simulink library "PhD_Library"  (R2018a)
settings: Solver=VariableStepAuto  StartTime=0.0  StopTime=10.0  RelTol=1e-3
values from neighbouring files (symbols this model uses):
  Ts = Ts_c    (= 1e-07)    [PlantStateEquations_abc_Script.m]
undefined symbols (not defined in the file or in its folder): D1, Delta, DiscIntNeverNeededParam, ESS, f_LPF_noise, fcutouti, fcutoutv, fn, fsw, Iap, Kp, PCC, Sn, tctrl, Ti, Ts_control, Ts_PWM, Uabp, Uanp, WT, X, zeta
libraries: $bdroot x84, powerlib_meascontrol x59, powerlib x56, peTransforms x32, cstblocks x2, simulink x2
(part 5 of 5)

== matlab function PhD_Library/Offshore_Oil_and_Wind/digital_ramp_gen/MATLAB Function ==
  data: up input; down input; rate input; y output; max input; min input; force input; forceval input; Ts input
%%%%%%%%%%%%%%%%%%%%%%%%%%%%%%%%%%%%%%%%%%%%%%%%%%%%%%%%%%%%%%%%%%%%%%%%%%
% Digital integrator
%%%%%%%%%%%%%%%%%%%%%%%%%%%%%%%%%%%%%%%%%%%%%%%%%%%%%%%%%%%%%%%%%%%%%%%%%%\
% Forward Euler method: as in matlab help
%   y(n) = y(n-1) + Ts(n-1)*x(n-1)
%   uset it to avoid algebraic loops

% All inputs are stored in states, so there is no direct feedthrough
% GAMBIARRA for avoiding algebraic loops
% see: https://www.mathworks.com/help/simulink/ug/integration-considerations-for-matlab-function-blocks.html

% Inputs
%   up: ramps up
%   down: ramps down (if both up and down, than stops)
%   max: max value for ramp
%   min: min value for ramp
%   force: if=1 sets integrator to forceval
%   forceval: see line above (max and min are respected
%   Ts: sampling time
% Output
%   y: output of the ramp

%%%%%%%%%%%%%%%%%%%%%%%%%%%%%%%%%%%%%%%%%%%%%%%%%%%%%%%%%%%%%%%%%%%%%%%%%%\
% Prog/rev history
%   Mota - 2021-05-21: first release

function y = DigRamp(up, down, rate, max, min, force, forceval, Ts)

% The value of the integrator
persistent i
persistent old_up
persistent old_down
persistent old_rate
persistent old_max
persistent old_min
persistent old_force
persistent old_forceval
persistent old_Ts

% Only at first cycle - outputs zero
if isempty(i)
    y = 0;
    i = 0;
    old_up = 0;
    old_down = 0;
    old_rate = 0;
    old_max = 0;
    old_min = 0;
    old_force = 0;
    old_forceval = 0;
    old_Ts = 0;
    % On the second cycle, output will still be zero, due to choices above
    return;
end

% auxiliary value
aux = 0;

% Bypassing the integrator with a value (can be used for followup)
if old_force == 1
    aux = old_forceval;
else
    %if not bypass, then calculate the next value of the integrator
    aux = i + old_Ts*old_rate*old_up + old_Ts*old_rate*old_down ;
end

%Limiting the integrator
if aux > old_max
    % max value has priority, i.e.,
    % if "max" is below "min" due to engineer error
    % the integrator will stop at "max"
    aux = old_max;
elseif aux < old_min
    % if integrator would cross the min, it will be stopped at min
    aux = old_min;
end

% output of the integrator
y = aux;

%update states
i = aux;
old_rate = rate;
%ramps up if up > 0
if up > 0
    old_up = 1;
else
    old_up = 0;
end
%ramps down if down > 0
if down > 0 
    old_down = -1;
else
    old_down = 0;
end
old_max = max;
old_min = min;
old_force = force;
old_forceval = forceval;
old_Ts = Ts;

== matlab function PhD_Library/Offshore_Oil_and_Wind/SR_Sini_Sdom/MATLAB Function ==
  data: S input; Q output; R input; Qbar output
%%%%%%%%%%%%%%%%%%%%%%%%%%%%%%%%%%%%%%%%%%%%%%%%%%%%%%%%%%%%%%%%%%%%%%%%%%
% Set Reset Flip Flop, Initial State Set, Set Dominant
%%%%%%%%%%%%%%%%%%%%%%%%%%%%%%%%%%%%%%%%%%%%%%%%%%%%%%%%%%%%%%%%%%%%%%%%%%\
% All inputs are stored in states, so there is no direct feedthrough
% GAMBIARRA for avoiding algebraic loops
% see: https://www.mathworks.com/help/simulink/ug/integration-considerations-for-matlab-function-blocks.html

% Inputs
%   set: if >0 set (dominant)
%   reset: if >0 reset
% Output
%   Q: 1 if set, 0 if reset
%   Q_bar: 0 if set, 1 if reset

%%%%%%%%%%%%%%%%%%%%%%%%%%%%%%%%%%%%%%%%%%%%%%%%%%%%%%%%%%%%%%%%%%%%%%%%%%\
% Prog/rev history
%   Mota - 2021-06-02: first release

function [Q,Qbar] = SR_Sini_Sdom(S, R)

persistent flipflop
persistent old_S
persistent old_R

% Only at first cycle - outputs zero
if isempty(flipflop)
    Q = 1;
    Qbar = 0;
    flipflop = 1;
    old_S = S;
    old_R = R;
    return;
end

if old_S >= 0
    Q = 1;
    Qbar = 0;
    flipflop = 1;
    return;
elseif old_R >= 0
    Q = 0;
    Qbar = 1;
    flipflop = 0;
    return;
else
    if flipflop == 0
        Q = 1;
        Qbar = 0;
    else
        Q = 0;
        Qbar = 1;
    end
end

old_S = S;
old_R = R;

== matlab function PhD_Library/Offshore_Oil_and_Wind/SR_Rini_Sdom/MATLAB Function ==
  data: S input; Q output; R input; Qbar output
%%%%%%%%%%%%%%%%%%%%%%%%%%%%%%%%%%%%%%%%%%%%%%%%%%%%%%%%%%%%%%%%%%%%%%%%%%
% Set Reset Flip Flop, Initial State Set, Set Dominant
%%%%%%%%%%%%%%%%%%%%%%%%%%%%%%%%%%%%%%%%%%%%%%%%%%%%%%%%%%%%%%%%%%%%%%%%%%\
% All inputs are stored in states, so there is no direct feedthrough
% GAMBIARRA for avoiding algebraic loops
% see: https://www.mathworks.com/help/simulink/ug/integration-considerations-for-matlab-function-blocks.html

% Inputs
%   set: if >0 set (dominant)
%   reset: if >0 reset
% Output
%   Q: 1 if set, 0 if reset
%   Q_bar: 0 if set, 1 if reset

%%%%%%%%%%%%%%%%%%%%%%%%%%%%%%%%%%%%%%%%%%%%%%%%%%%%%%%%%%%%%%%%%%%%%%%%%%\
% Prog/rev history
%   Mota - 2021-06-02: first release

function [Q,Qbar] = SR_Sini_Sdom(S, R)

persistent flipflop
persistent old_S
persistent old_R

% Only at first cycle - outputs zero
if isempty(flipflop)
    Q = 1;
    Qbar = 0;
    flipflop = 1;
    old_S = S;
    old_R = R;
    return;
end

if old_S >= 0
    Q = 1;
    Qbar = 0;
    flipflop = 1;
    return;
elseif old_R >= 0
    Q = 0;
    Qbar = 1;
    flipflop = 0;
    return;
else
    if flipflop == 0
        Q = 1;
        Qbar = 0;
    else
        Q = 0;
        Qbar = 1;
    end
end

old_S = S;
old_R = R;

== matlab function PhD_Library/Offshore_Oil_and_Wind/Enabled/MATLAB Function ==
  data: En input; Enabled output; Disabled output
%%%%%%%%%%%%%%%%%%%%%%%%%%%%%%%%%%%%%%%%%%%%%%%%%%%%%%%%%%%%%%%%%%%%%%%%%%
% Enabled block
%%%%%%%%%%%%%%%%%%%%%%%%%%%%%%%%%%%%%%%%%%%%%%%%%%%%%%%%%%%%%%%%%%%%%%%%%%\

% Inputs
%   Enabled: if >0 enabled
% Output
%   Enabled: 1 if enabled, 0 if disabled
%   Disabled: 1 if disabled, 0 if enabled

%%%%%%%%%%%%%%%%%%%%%%%%%%%%%%%%%%%%%%%%%%%%%%%%%%%%%%%%%%%%%%%%%%%%%%%%%%\
% Prog/rev history
%   Mota - 2021-06-02: first release

function [Enabled,Disabled] = Enabled(En)

if En > 0
    Enabled = 1;
    Disabled = 0;
else
    Enabled = 0;
    Disabled = 1;
end

== matlab function PhD_Library/Offshore_Oil_and_Wind/Storage/MATLAB Function ==
  data: x input; y output; store input
%%%%%%%%%%%%%%%%%%%%%%%%%%%%%%%%%%%%%%%%%%%%%%%%%%%%%%%%%%%%%%%%%%%%%%%%%%
% Storage block
%%%%%%%%%%%%%%%%%%%%%%%%%%%%%%%%%%%%%%%%%%%%%%%%%%%%%%%%%%%%%%%%%%%%%%%%%%\

% Inputs
%   Store: if > 0 store input
%   x = input
% Output
%   y = output

%%%%%%%%%%%%%%%%%%%%%%%%%%%%%%%%%%%%%%%%%%%%%%%%%%%%%%%%%%%%%%%%%%%%%%%%%%\
% Prog/rev history
%   Mota - 2021-06-02: first release

function y  = Store(x, store)

persistent dado

if isempty(dado)
    dado = 0;
end

if store <= 0
    y = dado;
    return
else
    y = x;
    dado = x;
end
